simulink model "adptive_3DOF"  (R2020b)
settings: Solver=VariableStepAuto  StartTime=0.0  StopTime=10  RelTol=1e-3
model workspace (MAT data in the model file):
  A = 0.785398163397
  G1 = 27.1997755633
  G2 = 12
  G3 = -6.75
  I = 1.38360428917
  I1x = 0.0001
  I1y = 0.0001
  I1z = 0.0001
  I2x = 0.0001
  I2y = 0.0001
  I2z = 0.0001
  I3x = 0.0001
  I3y = 0.0001
  I3z = 0.0001
  I_com = 514.351036867
  L1 = 1
  L2 = 0.8
  L3 = 0.5
  gam1 = 0.05
  gam2 = 0.3
  gam3 = 0.1
  ka = 0.1
  kp1 = 1.5
  kp2 = 20
  kp3 = 1
  kv1 = 0.2
  kv2 = 0.2
  kv3 = 0.2
  m1 = 1
  m2 = 0.7
  m3 = 0.45
  omega = 0.5
  t = 0
  tau = 5
  tf = 3
  the1 = 0.959931088597
  the2 = -0.959931088597
  the3 = 0.2
  theta1 = 0.959931088597
  theta2 = -0.959931088597
  theta3 = 0.2
  tick = 0.02
  ts = 0
settings Model: Creator=lamth  LastModifiedBy=lamth

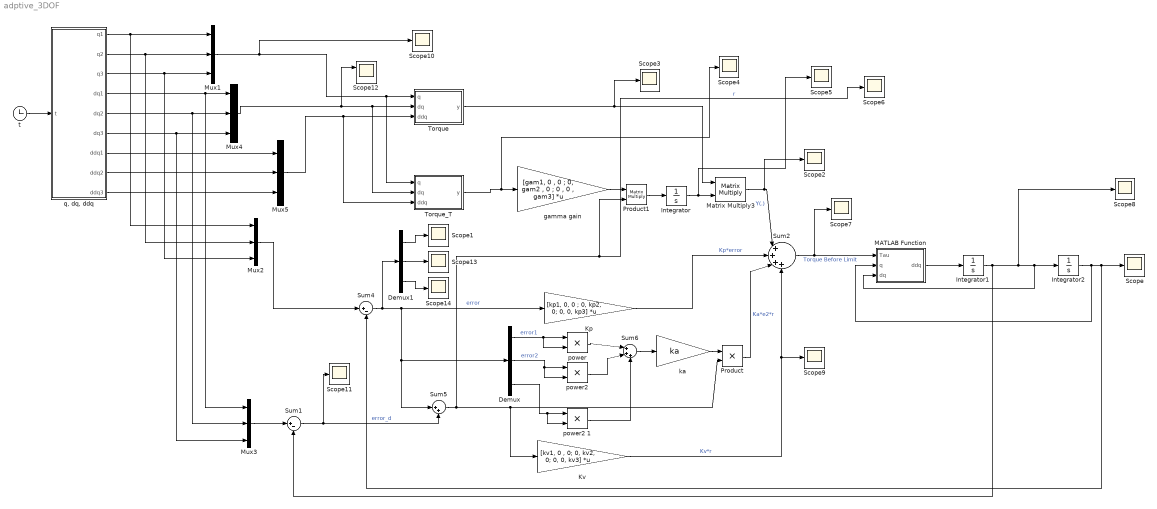
== system adptive_3DOF ==
  Demux : Demux  Outputs=3
  Demux1 : Demux  Outputs=3
  Integrator : Integrator
  Integrator1 : Integrator
  Integrator2 : Integrator
  Kp : Gain  Gain=[kp1, 0, 0 ; 0, kp2, 0; 0, 0, kp3]  Multiplication=Matrix(K*u)
  Kv : Gain  Gain=[kv1, 0 , 0; 0, kv2, 0; 0, 0, kv3]  Multiplication=Matrix(K*u)
  MATLAB Function : MATLAB Function  TreatAsAtomicUnit=on
  Matrix Multiply3 : Product  Multiplication=Matrix(*)
  Mux{1..5} (5 alike) : Mux  Inputs=3
  Product : Product
  Product1 : Product  Multiplication=Matrix(*)
  Scope{,1..11,13..14} (14 alike) : Scope
  Scope12 : Scope  NumInputPorts=2
  Sum1 : Sum  Inputs=|+-
  Sum2 : Sum  Inputs=|++++
  Sum4 : Sum  Inputs=|+-
  Sum5 : Sum  Inputs=|++
  Sum6 : Sum  Inputs=|+++
  Torque : MATLAB Function  TreatAsAtomicUnit=on
  Torque_T : MATLAB Function  TreatAsAtomicUnit=on
  gamma gain : Gain  Gain=[gam1, 0 , 0 ; 0, gam2 , 0 ; 0 , 0 , gam3]  Multiplication=Matrix(K*u)
  ka : Gain  Gain=ka
  power : Product
  "power2 " : Product
  power2 1 : Product
  "q, dq, ddq" : MATLAB Function  TreatAsAtomicUnit=on
  t : Clock
  wires:
  Mux3/1 -> Sum1/1
  Sum4/1 -> Sum5/1, Demux/1, Kp/1, Demux1/1  "error"
  Demux/2 -> "power2 "/2, "power2 "/1  "error2"
  Matrix Multiply3/1 -> Scope2/1, Sum2/1  "Y(.)"
  Sum5/1 -> Scope6/1, Product1/2, Kv/1, Product/2  "r"
  Kv/1 -> Scope9/1, Sum2/4  "Kv*r"
  power/1 -> Sum6/1
  Kp/1 -> Sum2/2  "Kp*error"
  "power2 "/1 -> Sum6/2
  Sum6/1 -> ka/1
  Sum1/1 -> Sum5/2, Scope11/1  "error_d"
  Mux2/1 -> Sum4/1
  Product/1 -> Sum2/3  "Ka*e2*r"
  ka/1 -> Product/1
  Demux/1 -> power/2, power/1  "error1"
  Torque_T/1(y) -> Scope4/1, gamma gain/1
  Torque/1(y) -> Scope3/1, Matrix Multiply3/1
  gamma gain/1 -> Product1/1
  Product1/1 -> Integrator/1
  Integrator/1 -> Scope5/1, Matrix Multiply3/2
  Demux/3 -> power2 1/2, power2 1/1
  power2 1/1 -> Sum6/3
  MATLAB Function/1(ddq) -> Integrator1/1
  Integrator1/1 -> Integrator2/1, MATLAB Function/3(dq), Scope8/1, Sum1/2
  t/1 -> "q, dq, ddq"/1(t)
  "q, dq, ddq"/1(q1) -> Mux1/1, Mux2/1
  "q, dq, ddq"/2(q2) -> Mux2/2, Mux1/2
  "q, dq, ddq"/3(q3) -> Mux2/3, Mux1/3
  "q, dq, ddq"/4(dq1) -> Mux3/1, Mux4/1
  "q, dq, ddq"/5(dq2) -> Mux3/2, Mux4/2
  "q, dq, ddq"/6(dq3) -> Mux3/3, Mux4/3
  "q, dq, ddq"/7(ddq1) -> Mux5/1
  "q, dq, ddq"/8(ddq2) -> Mux5/2
  "q, dq, ddq"/9(ddq3) -> Mux5/3
  Mux1/1 -> Scope10/1, Torque_T/1(q), Torque/1(q)
  Mux4/1 -> Torque_T/2(dq), Torque/2(dq), Scope12/1
  Mux5/1 -> Torque_T/3(ddq), Torque/3(ddq)
  Integrator2/1 -> Scope/1, Sum4/2, MATLAB Function/2(q)
  Sum2/1 -> MATLAB Function/1(Tau), Scope7/1  "Torque Before Limit"
  Demux1/1 -> Scope1/1
  Demux1/2 -> Scope13/1
  Demux1/3 -> Scope14/1

== matlab function adptive_3DOF/MATLAB Function ==
  data: Tau input; ddq output; q input; dq input
function ddq  = fcn(Tau,q,dq)
[m1,m2,m3,L1,L2,L3,I1x,I1y,I1z,I2x,I2y,I2z,I3x,I3y,I3z]=parameter ();

q=zeros(3,1);
dq=zeros(3,1);

% Khai bao ma tran khoi luong M
M=zeros(3,3);
M(1,1)= (9/4)*m1*L1^2+I1z+3*m2*L2*L1*cos(q(2))+L1^2*m2+(9/4)*m2*L2^2+I2y+2*m3*L2*L1*cos(q(2))+3*m3*L1*q(3)*sin(q(2))+L1^2*m3+L2^2*m3+(9/4)*m3*q(3)^2+I3y;
M(1,2)= (3/2)*m2*L2*L1*cos(q(2))+(9/4)*m2*L2^2+I2y+m3*L2*L1*cos(q(2))+(3/2)*m3*L1*q(3)*sin(q(2))+L2^2*m3+(9/4)*m3*q(3)^2+I3y;
M(1,3)= -(3/2)*L1*m3*cos(q(2))-(3/2)*L2*m3;


M(2,1)=(3/2)*m2*L2*L1*cos(q(2))+(9/4)*m2*L2^2+I2y+m3*L2*L1*cos(q(2))+(3/2)*m3*L1*q(3)*sin(q(2))+L2^2*m3+(9/4)*m3*q(3)^2+I3y;
M(2,2)=(9/4)*m2*L2^2+I2y+L2^2*m3+(9/4)*m3*q(3)^2+I3y;
M(2,3)=-(3/2)*L2*m3;

M(3,1)=-(3/2)*L1*m3*cos(q(2))-(3/2)*L2*m3;
M(3,2)=-(3/2)*L2*m3;
M(3,3)=(9/4)*m3;

% Khai bao ma tran Coriolis C
%h=-m2*L1*Lc2*sin(q(2));
Co=zeros(3,3);
Co(1,1)=-3*L1*L2*sin(q(2))*dq(2)*m2-2*L1*L2*sin(q(2))*dq(2)*m3+3*L1*cos(q(2))*dq(2)*m3*q(3)+3*L1*m3*sin(q(2))*dq(3)+(9/2)*m3*q(3)*dq(3);
Co(1,2)=-(3/2)*L1*L2*sin(q(2))*dq(2)*m2-L1*L2*sin(q(2))*dq(2)*m3+(3/2)*L1*cos(q(2))*dq(2)*m3*q(3)+(3/2)*L1*m3*sin(q(2))*dq(3)+(9/2)*m3*q(3)*dq(3);
Co(1,3)=(3/2)*L1*m3*sin(q(2))*dq(2);


Co(2,1)=(3/2)*L1*L2*sin(q(2))*dq(1)*m2+L1*L2*sin(q(2))*dq(1)*m3-(3/4)*L1*L2*sin(q(2))*dq(2)*m2-(1/2)*L1*L2*sin(q(2))*dq(2)*m3-(3/2)*L1*cos(q(2))*dq(1)*m3*q(3)+(3/4)*L1*cos(q(2))*dq(2)*m3*q(3)+(3/4)*L1*m3*sin(q(2))*dq(3)+(9/2)*m3*q(3)*dq(3);
Co(2,2)=(3/4)*L1*L2*sin(q(2))*dq(1)*m2+(1/2)*L1*L2*sin(q(2))*dq(1)*m3-(3/4)*L1*cos(q(2))*dq(1)*m3*q(3)+(9/2)*m3*q(3)*dq(3);
Co(2,3)=-(3/4)*L1*m3*sin(q(2))*dq(1);


Co(3,1)=-(3/2)*L1*m3*sin(q(2))*dq(1)+(3/4)*L1*m3*sin(q(2))*dq(2)-(9/4)*dq(1)*m3*q(3)-(9/4)*m3*q(3)*dq(2);
Co(3,2)=-(3/4)*L1*m3*sin(q(2))*dq(1)-(9/4)*dq(1)*m3*q(3)-(9/4)*m3*q(3)*dq(2);
Co(3,3)=0;

% Ma tran the nang hap dan
G=zeros(3,1);
G(1,1)=15*m1*L1*cos(q(1))+10*m2*L1*cos(q(1))+10*m3*L1*cos(q(1))+15*m2*L2*cos(q(1)+q(2))+10*m3*L2*cos(q(1)+q(2))+15*m3*sin(q(1)+q(2))*q(3);
G(2,1)=15*m2*L2*cos(q(1)+q(2))+10*m3*L2*cos(q(1)+q(2))+15*m3*sin(q(1)+q(2))*q(3);
G(3,1)=-15*m3*cos(q(1)+q(2));


% Pt DLH
ddq=inv(M)*(Tau-Co*dq-G);

== matlab function adptive_3DOF/Torque_T ==
  data: q input; y output; dq input; ddq input
function y = Tau_T(q,dq,ddq)

[m1,m2,m3,L1,L2,L3,I1x,I1y,I1z,I2x,I2y,I2z,I3x,I3y,I3z,g]=parameter ();


Y11=L1 * (L1 * ddq(1) + cos(q(1)) * g);
Y12=g * L2 * cos(q(1) + q(2)) + 0.2e1 * dq(2) * L2 * L1 * (dq(1) + dq(2) / 0.2e1) * sin(q(2)) + 0.2e1 * L1 * L2 * cos(q(2)) * ddq(1) + g * L1 * cos(q(1)) + L1 ^ 2 * ddq(1) + L1 * L2 * ddq(2) + L2 ^ 2 * ddq(1);
Y13=-L1 * (2 * dq(1) * q(3) + ddq(3)) * cos((2 * q(1) + q(2))) + L1 * dq(3) * (dq(2) + 1) * sin((2 * q(1) + q(2))) + g * L2 * cos((q(1) + q(2))) - g * q(3) * sin((q(1) + q(2))) + 0.2e1 * (dq(1) + dq(2) / 0.2e1) * L1 * (L2 * dq(2) + q(3)) * sin(q(2)) + 0.2e1 * L1 * L2 * cos(q(2)) * ddq(1) + g * L1 * cos(q(1)) + L1 ^ 2 * ddq(1) + L2 ^ 2 * ddq(1) + L1 * L2 * ddq(2) + ddq(1) * q(3) - L2 * ddq(3);

Y21=0;
Y22=(g * cos(q(1) + q(2)) + L1 * dq(1) * (dq(1) + dq(2) - 1) * sin(q(2)) + L1 * ddq(1) + L2 * (ddq(1) + ddq(2))) * L2;
Y23=-L1 * cos((2 * q(1) + q(2))) * dq(1) * q(3) - L1 * sin((2 * q(1) + q(2))) * dq(1) * dq(3) + g * L2 * cos((q(1) + q(2))) + g * q(3) * sin((q(1) + q(2))) + L1 * L2 * dq(1) * (dq(1) + dq(2) - 0.1e1) * sin(q(2)) + (ddq(1) + ddq(2)) * L2 ^ 2 + (L1 * ddq(1) - ddq(3)) * L2 + q(3) * (ddq(1) + ddq(2));

Y31=0;
Y32=0;
Y33=0.2e1 * (dq(1) + dq(2) / 0.2e1 - 0.1e1 / 0.2e1) * dq(1) * L1 * sin((2 * q(1) + q(2))) - L1 * (ddq(1) + ddq(2)) * cos((2 * q(1) + q(2))) - g * cos((q(1) + q(2))) - ddq(1) * L2 - L2 * ddq(2) - dq(1) ^ 2 / 0.2e1 - dq(1) * dq(2) - dq(2) ^ 2 / 0.2e1 + ddq(3);

% Pt DLH
y = [Y11 Y21 Y31; Y12 Y22 Y32; Y13 Y23 Y33];

== matlab function adptive_3DOF/q, dq, ddq ==
  data: q1 output; t input; q2 output; q3 output; dq1 output; dq2 output; dq3 output; ddq1 output; ddq2 output; ddq3 output
function [q1,q2,q3,dq1,dq2,dq3,ddq1,ddq2,ddq3] = fcn(t)
pi=3.14;
q1 = sin(t*10^-5);
q2 = cos(t*10^-6);
q3 = -sin(t*10^-6);

dq1=(10^-5)*cos(t*10^-5);
dq2=-(10^-4)*sin(t*10^-6);
dq3=-(10^-6)*cos(t*10^-6);

ddq1=-(10^-5)*(10^-5)*sin(t*10^-5);
ddq2=-(10^-6)*(10^-6)*cos(t*10^-6);
ddq3=(10^-6)*(10^-5)*sin(t*10^-6);

== matlab function adptive_3DOF/Torque ==
  data: q input; y output; dq input; ddq input
function y = Tau(q,dq,ddq)

[m1,m2,m3,L1,L2,L3,I1x,I1y,I1z,I2x,I2y,I2z,I3x,I3y,I3z,g]=parameter ();


Y11=0.15e2 * L1 * cos(q(1)) + 0.9e1 / 0.4e1 * L1 ^ 2 * ddq(1);
Y12=0.3e1 * L2 * (0.5e1 * cos(q(1)) + L1 * (ddq(1) + ddq(2) / 0.2e1)) * cos(q(2)) - 0.3e1 * L2 * (0.5e1 * sin(q(1)) + L1 * dq(2) * (dq(1) + dq(2) / 0.2e1)) * sin(q(2)) + 0.10e2 * L1 * cos(q(1)) + (0.9e1 * ddq(1) + 0.9e1 * ddq(2)) * L2 ^ 2 / 0.4e1 + L1 ^ 2 * ddq(1);
Y13=(0.60e2 * cos(q(1)) * q(3) - 0.40e2 * L2 * sin(q(1)) + 0.6e1 * L1 * ((2 * ddq(1) + ddq(2)) * q(3) - 0.4e1 / 0.3e1 * dq(2) * (dq(1) + dq(2) / 0.2e1) * L2 + 0.2e1 * dq(3) * (dq(1) + dq(2)))) * sin(q(2)) / 0.4e1 + (0.40e2 * L2 * cos(q(1)) + 0.60e2 * sin(q(1)) * q(3) + 0.4e1 * (0.3e1 * dq(2) * (dq(1) + dq(2) / 0.2e1) * q(3) + (2 * ddq(1) + ddq(2)) * L2 - 0.3e1 / 0.2e1 * ddq(3)) * L1) * cos(q(2)) / 0.4e1 + 0.10e2 * L1 * cos(q(1)) + L1 ^ 2 * ddq(1) + (9 * ddq(1) + 9 * ddq(2)) * q(3) ^ 2 / 0.4e1 + 0.9e1 / 0.2e1 * dq(3) * (dq(1) + dq(2)) * q(3) + ((ddq(1) + ddq(2)) * L2 - 0.3e1 / 0.2e1 * ddq(3)) * L2;


Y21=0;
Y22=0.3e1 / 0.2e1 * L2 * (0.10e2 * cos(q(1) + q(2)) + ddq(1) * L1 * cos(q(2)) + dq(1) ^ 2 * L1 * sin(q(2)) + 0.3e1 / 0.2e1 * (ddq(1) + ddq(2)) * L2);
Y23=0.10e2 * L2 * cos(q(1) + q(2)) + 0.15e2 * sin(q(1) + q(2)) * q(3) + (-0.6e1 * L1 * dq(1) ^ 2 * q(3) + 0.4e1 * L1 * L2 * ddq(1)) * cos(q(2)) / 0.4e1 + (0.4e1 * L1 * L2 * dq(1) ^ 2 + 0.6e1 * L1 * ddq(1) * q(3)) * sin(q(2)) / 0.4e1 + ((9 * ddq(2)) + 0.9e1 * ddq(1)) * q(3) ^ 2 / 0.4e1 + 0.9e1 / 0.2e1 * dq(3) * (dq(1) + dq(2)) * q(3) + ((ddq(1) + ddq(2)) * L2 - 0.3e1 / 0.2e1 * ddq(3)) * L2;


Y31=0;
Y32=0;
Y33=-0.3e1 / 0.2e1 * dq(1) ^ 2 * L1 * sin(q(2)) - 0.3e1 / 0.2e1 * ddq(1) * L1 * cos(q(2)) - 0.9e1 / 0.4e1 * dq(1) ^ 2 * q(3) - 0.9e1 / 0.2e1 * dq(1) * q(3) * dq(2) - 0.9e1 / 0.4e1 * dq(2) ^ 2 * q(3) - 0.3e1 / 0.2e1 * L2 * ddq(2) - 0.3e1 / 0.2e1 * ddq(1) * L2 + 0.9e1 / 0.4e1 * ddq(3) - 0.15e2 * cos(q(1) + q(2));


% Pt DLH
y = [Y11 Y12 Y13; Y21 Y22 Y23; Y31 Y32 Y33];
